simulink model "Modelo5_1_2_C_1"  (R2020a)
settings: Solver=VariableStepAuto  StartTime=0.0  StopTime=10.0  RelTol=1e-3
values from neighbouring files (symbols this model uses):
  b_eq = b_m + b_l/(r^2)    (= 2.19444444444e-05)    [LTI_vs_LPV_vs_NL_realimentado.m]    (also in Modelo_linealizado.m)
  C_ts = 0.818    [LTI_vs_LPV_vs_NL_realimentado.m]    (also in Modelo_linealizado.m)
  J_eq = J_m + J_l/(r^2)    (= 1.97847222222e-05)    [LTI_vs_LPV_vs_NL_realimentado.m]    (also in Modelo_linealizado.m)
  L_d = 6.6/1000    (= 0.0066)    [Curvas_carc.m]    (also in LTI_vs_LPV_vs_NL_realimentado.m; Modelo_linealizado.m)
  L_ls = 0.8/1000    (= 0.0008)    [LTI_vs_LPV_vs_NL_realimentado.m]    (also in Modelo_linealizado.m)
  L_q = 5.8/1000    (= 0.0058)    [Curvas_carc.m]    (also in LTI_vs_LPV_vs_NL_realimentado.m; Modelo_linealizado.m = -R_s/z)
  lambda_m = 0.01546    [Curvas_carc.m]    (also in LTI_vs_LPV_vs_NL_realimentado.m = 0.016; Modelo_linealizado.m = 0.016)
  Pp = 3    [AnalisisDeEstabilidad.m]    (also in LTI_vs_LPV_vs_NL_realimentado.m; Modelo_linealizado.m; parametros.m)
  r = 120    [AnalisisDeEstabilidad.m]    (also in LTI_vs_LPV_vs_NL_realimentado.m; Modelo_linealizado.m; parametros.m)
  R_s = 1.02    [Curvas_carc.m]    (also in LTI_vs_LPV_vs_NL_realimentado.m = R_s_o; Modelo_linealizado.m = R_s_o)
  R_ts_amb = 146.7    [LTI_vs_LPV_vs_NL_realimentado.m]    (also in Modelo_linealizado.m)
settings Model: Creator=matie  LastModifiedBy=Juan

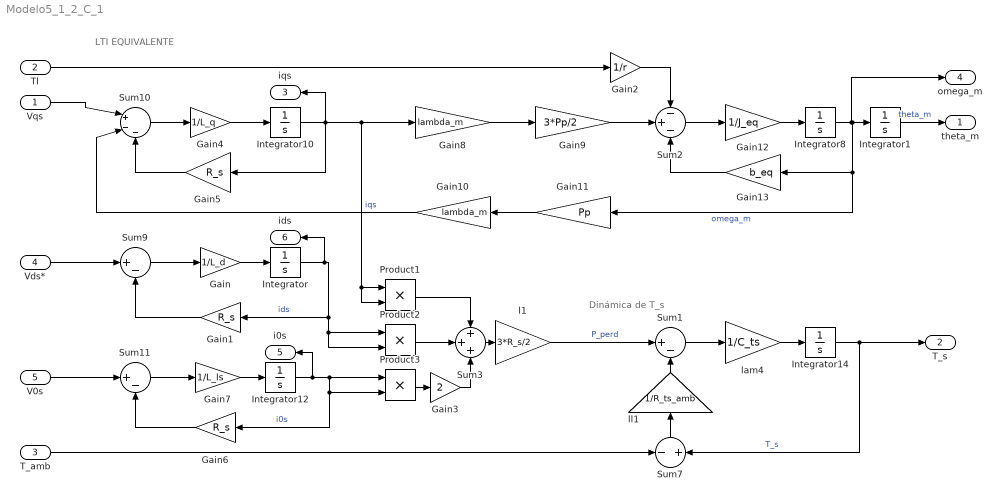
== system Modelo5_1_2_C_1 ==
  note: LTI EQUIVALENTE
  note: Dinámica de T_s
  Vqs : Inport
  Tl : Inport  Port=2
  T_amb : Inport  Port=3
  Vds* : Inport  Port=4
  V0s : Inport  Port=5
  Gain : Gain  Gain=1/L_d
  Gain1 : Gain  Gain=R_s
  Gain10 : Gain  Gain=lambda_m
  Gain11 : Gain  Gain=Pp
  Gain12 : Gain  Gain=1/J_eq
  Gain13 : Gain  Gain=b_eq
  Gain2 : Gain  Gain=1/r
  Gain3 : Gain  Gain=2
  Gain4 : Gain  Gain=1/L_q
  Gain5 : Gain  Gain=R_s
  Gain6 : Gain  Gain=R_s
  Gain7 : Gain  Gain=1/L_ls
  Gain8 : Gain  Gain=lambda_m
  Gain9 : Gain  Gain=3*Pp/2
  Integrator{,1,8,10,12,14} (6 alike) : Integrator
  Product1 : Product
  Product2 : Product
  Product3 : Product
  Sum1 : Sum  Inputs=|+-
  Sum10 : Sum  Inputs=|+--
  Sum11 : Sum  Inputs=|+-
  Sum2 : Sum  Inputs=-+-
  Sum3 : Sum  Inputs=+++
  Sum7 : Sum  Inputs=-+
  Sum9 : Sum  Inputs=|+-
  l1 : Gain  Gain=3*R_s/2
  lam4 : Gain  Gain=1/C_ts
  ll1 : Gain  Gain=1/R_ts_amb
  theta_m : Outport
  T_s : Outport  Port=2
  iqs : Outport  Port=3
  omega_m : Outport  Port=4
  i0s : Outport  Port=5
  ids : Outport  Port=6
  wires:
  ll1/1 -> Sum1/2
  T_amb/1 -> Sum7/1
  l1/1 -> Sum1/1  "P_perd"
  Gain2/1 -> Sum2/1
  Gain12/1 -> Integrator8/1
  Gain13/1 -> Sum2/3
  Gain8/1 -> Gain9/1
  Sum2/1 -> Gain12/1
  Gain4/1 -> Integrator10/1
  Gain11/1 -> Gain10/1
  Gain9/1 -> Sum2/2
  Sum10/1 -> Gain4/1
  lam4/1 -> Integrator14/1
  Integrator14/1 -> Sum7/2, T_s/1  "T_s"
  Gain5/1 -> Sum10/3
  Sum1/1 -> lam4/1
  Tl/1 -> Gain2/1
  Vqs/1 -> Sum10/1
  Gain10/1 -> Sum10/2
  Integrator10/1 -> Product1/2, Product1/1, Gain8/1, Gain5/1, iqs/1  "iqs"
  Sum7/1 -> ll1/1
  Integrator8/1 -> omega_m/1, Integrator1/1, Gain11/1, Gain13/1  "omega_m"
  Integrator1/1 -> theta_m/1  "theta_m"
  Gain1/1 -> Sum9/2
  Sum9/1 -> Gain/1
  Gain6/1 -> Sum11/2
  Integrator12/1 -> Product3/1, Product3/2, Gain6/1, i0s/1  "i0s"
  Gain/1 -> Integrator/1
  Sum11/1 -> Gain7/1
  V0s/1 -> Sum11/1
  Vds*/1 -> Sum9/1
  Gain7/1 -> Integrator12/1
  Sum3/1 -> l1/1
  Product2/1 -> Sum3/2
  Product1/1 -> Sum3/1
  Integrator/1 -> Gain1/1, Product2/2, Product2/1, ids/1  "ids"
  Product3/1 -> Gain3/1
  Gain3/1 -> Sum3/3
